simulink model "Helicopter_Sim"  (Simulink 8.6)
settings: Solver=ode4  StartTime=0.0  StopTime=Simulation_Tmax  FixedStep=Simulation_DT  RelTol=1e-3
values from neighbouring files (symbols this model uses):
  Disturbance_mass = 0    [Helicopter_EqPts.m]    (also in Helicopter_Params.m = 70)
  gravity = 9.81    [Helicopter_EqPts.m]    (also in Helicopter_Params.m)
  Helicopter_Fuselage_Area = 2    [Helicopter_EqPts.m]    (also in Helicopter_Params.m = 200)
  Helicopter_Fuselage_DragCoefficient = 15    [Helicopter_EqPts.m]    (also in Helicopter_Params.m = 40)
  Helicopter_Fuselage_Mass = 5    [Helicopter_EqPts.m]    (also in Helicopter_Params.m = 1000)
  Helicopter_Fuselage_RotInertia = 50    [Helicopter_EqPts.m]    (also in Helicopter_Params.m = 5)
  Helicopter_mRotor_Area = pi*Helicopter_mRotor_Radius^2    (= 3.14159265359)    [Helicopter_EqPts.m]    (also in Helicopter_Params.m = 314.159265359)
  Helicopter_mRotor_Ib = 10    [Helicopter_EqPts.m]    (also in Helicopter_Params.m)
  Helicopter_mRotor_Omega = 10    [Helicopter_EqPts.m]    (also in Helicopter_Params.m)
  Helicopter_mRotor_Radius = 1    [Helicopter_EqPts.m]    (also in Helicopter_Params.m = 10)
  Helicopter_N = 3    [Helicopter_EqPts.m]    (also in Helicopter_Params.m)
  Helicopter_tDistance = 3    [Helicopter_EqPts.m]    (also in Helicopter_Params.m = 20)
  Helicopter_tRotor_Area = pi*Helicopter_tRotor_Radius^2    (= 0.785398163397)    [Helicopter_EqPts.m]    (also in Helicopter_Params.m = 7853.98163397)
  Helicopter_tRotor_Radius = 0.5    [Helicopter_EqPts.m]    (also in Helicopter_Params.m = 50)
  Omega_Tail = -0.002043    [Helicopter_Params.m]
  rho_air = 1.22    [Helicopter_EqPts.m]    (also in Helicopter_Params.m)
  Simulation_DT = 0.00125    [Helicopter_EqPts.m]    (also in Helicopter_Params.m = 0.0125)
  Theta = 0.001706    [Helicopter_Params.m]
settings Model: Creator=Dana  LastModifiedBy=dmartin_a
settings DataIOCC: ExternalInput=[Helicopter, Disturbance, Simulation, gravity, rho_air]  InitialState=[Initial.Z ;Initial.R;]  SignalLoggingSaveFormat=Dataset  ReturnWorkspaceOutputs=on
settings OptimizationCC: ExpressionDepthLimit=128
settings DebuggingCC: UnderspecifiedInitializationDetection=Simplified  MergeDetectMultiDrivingBlocksExec=error  SolverPrmCheckMsg=none  FcnCallInpInsideContextMsg=EnableAllAsError  StateNameClashWarn=none  InitInArrayFormatMsg=error
settings GRTTargetCC: CombineOutputUpdateFcns=on  GRTInterface=off

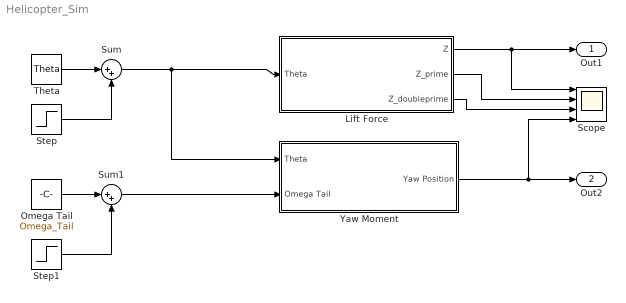
== system Helicopter_Sim ==
  Lift Force : Subsystem
  Omega Tail : Constant  Value=Omega_Tail  SampleTime=Simulation_DT
  Scope : Scope  NumInputPorts=4
  Step : Step  SampleTime=Simulation_DT
  Step1 : Step  SampleTime=Simulation_DT
  Sum : Sum  Inputs=|++
  Sum1 : Sum  Inputs=|++
  Theta : Constant  Value=Theta  SampleTime=Simulation_DT
  Yaw Moment : Subsystem
  Out1 : Outport
  Out2 : Outport  Port=2
  wires:
  Lift Force/1(Z) -> Scope/1, Out1/1
  Yaw Moment/1(Yaw Position) -> Scope/4, Out2/1
  Step/1 -> Sum/2
  Sum/1 -> Yaw Moment/1(Theta), Lift Force/1(Theta)
  Step1/1 -> Sum1/2
  Omega Tail/1 -> Sum1/1
  Sum1/1 -> Yaw Moment/2(Omega Tail)
  Theta/1 -> Sum/1
  Lift Force/2(Z_prime) -> Scope/2
  Lift Force/3(Z_doubleprime) -> Scope/3

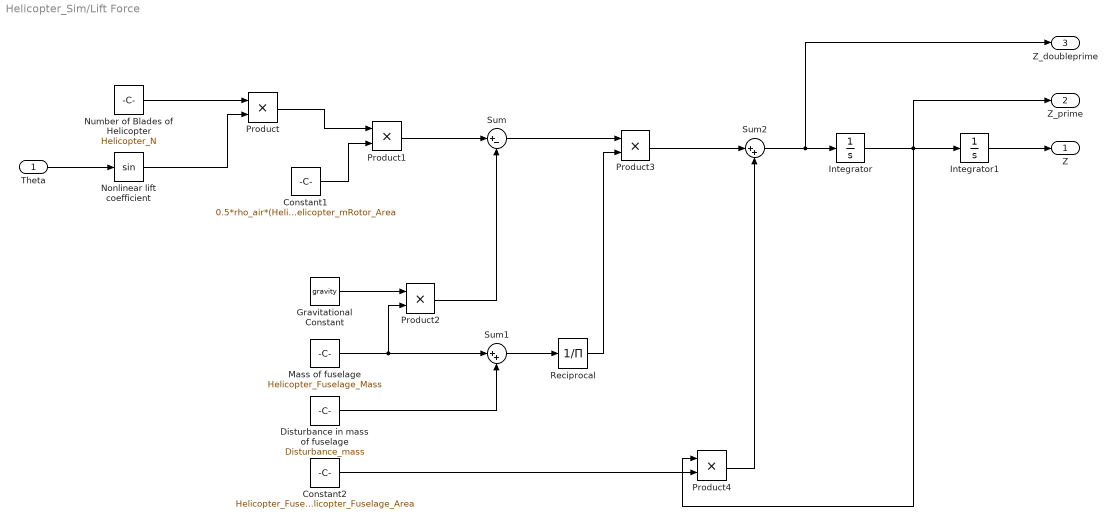
== system Helicopter_Sim/Lift Force ==
  Theta : Inport
  Constant1 : Constant  Value=0.5*rho_air*(Helicopter_mRotor_Omega*Helicopter_mRotor_Radius)^2*Helicopter_mRotor_Area  SampleTime=Simulation_DT
  Constant2 : Constant  Value=Helicopter_Fuselage_DragCoefficient*0.5*rho_air*Helicopter_Fuselage_Area  SampleTime=Simulation_DT
  Disturbance in mass of fuselage : Constant  Value=Disturbance_mass  SampleTime=Simulation_DT
  Gravitational Constant : Constant  Value=gravity  SampleTime=Simulation_DT
  Integrator : Integrator  LimitOutput=on  UpperSaturationLimit=20  LowerSaturationLimit=0
  Integrator1 : Integrator  LimitOutput=on  UpperSaturationLimit=20  LowerSaturationLimit=0
  Mass of fuselage : Constant  Value=Helicopter_Fuselage_Mass  SampleTime=Simulation_DT
  Nonlinear lift coefficient : Trigonometry  OutputSignalType=real
  Number of Blades of Helicopter : Constant  Value=Helicopter_N  SampleTime=Simulation_DT
  Product{,1..4} (5 alike) : Product
  Reciprocal : Product  Inputs=/  SaturateOnIntegerOverflow=on  RndMeth=Zero
  Sum : Sum  Inputs=|+-
  Sum1 : Sum  Inputs=|++
  Sum2 : Sum  Inputs=|++
  Z : Outport
  Z_prime : Outport  Port=2
  Z_doubleprime : Outport  Port=3
  wires:
  Theta/1 -> Nonlinear lift coefficient/1
  Number of Blades of Helicopter/1 -> Product/1
  Nonlinear lift coefficient/1 -> Product/2
  Product/1 -> Product1/1
  Constant1/1 -> Product1/2
  Mass of fuselage/1 -> Product2/2, Sum1/1
  Gravitational Constant/1 -> Product2/1
  Product2/1 -> Sum/2
  Product1/1 -> Sum/1
  Disturbance in mass of fuselage/1 -> Sum1/2
  Sum1/1 -> Reciprocal/1
  Reciprocal/1 -> Product3/2
  Sum/1 -> Product3/1
  Product3/1 -> Sum2/1
  Constant2/1 -> Product4/2
  Product4/1 -> Sum2/2
  Sum2/1 -> Z_doubleprime/1, Integrator/1
  Integrator/1 -> Z_prime/1, Integrator1/1, Product4/1
  Integrator1/1 -> Z/1

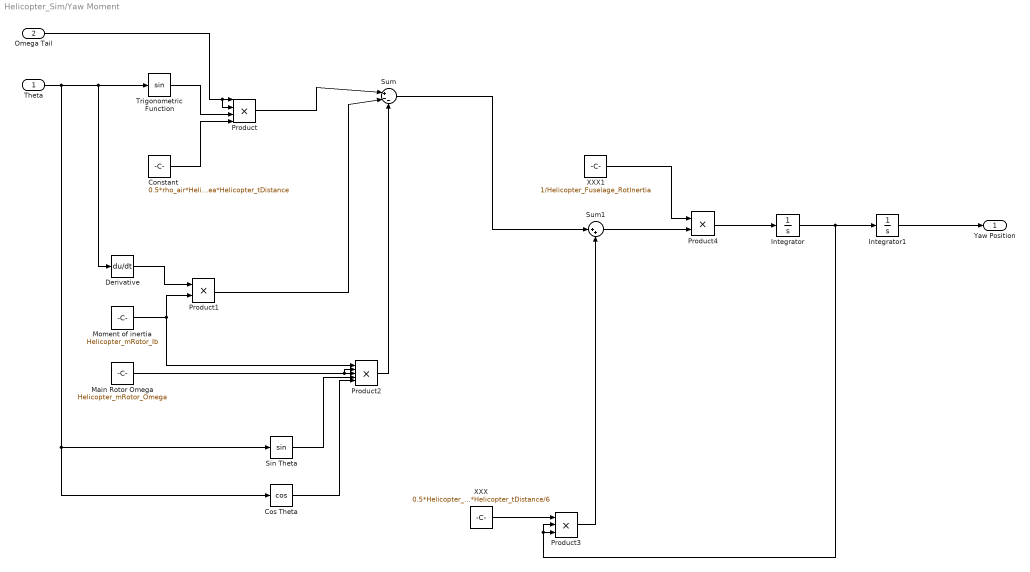
== system Helicopter_Sim/Yaw Moment ==
  Theta : Inport
  Omega Tail : Inport  Port=2
  Constant : Constant  Value=0.5*rho_air*Helicopter_tRotor_Radius^2*Helicopter_tRotor_Area*Helicopter_tDistance  SampleTime=Simulation_DT
  Cos Theta : Trigonometry  Operator=cos
  Derivative : Derivative
  Integrator : Integrator  LimitOutput=on  UpperSaturationLimit=20  LowerSaturationLimit=0
  Integrator1 : Integrator  LimitOutput=on  UpperSaturationLimit=20  LowerSaturationLimit=0
  Main Rotor Omega : Constant  Value=Helicopter_mRotor_Omega  SampleTime=Simulation_DT
  Moment of inertia : Constant  Value=Helicopter_mRotor_Ib  SampleTime=Simulation_DT
  Product : Product  Inputs=4
  Product1 : Product
  Product2 : Product  Inputs=5
  Product3 : Product  Inputs=3
  Product4 : Product
  Sin Theta : Trigonometry
  Sum : Sum  Inputs=|+--
  Sum1 : Sum  Inputs=|++
  Trigonometric Function : Trigonometry
  XXX : Constant  Value=0.5*Helicopter_Fuselage_DragCoefficient*rho_air*2*Helicopter_Fuselage_Area*Helicopter_tDistance/6  SampleTime=Simulation_DT
  XXX1 : Constant  Value=1/Helicopter_Fuselage_RotInertia  SampleTime=Simulation_DT
  Yaw Position : Outport
  wires:
  Theta/1 -> Cos Theta/1, Sin Theta/1, Derivative/1, Trigonometric Function/1
  Product/1 -> Sum/1
  Moment of inertia/1 -> Product1/2, Product2/1
  Derivative/1 -> Product1/1
  Product1/1 -> Sum/2
  Main Rotor Omega/1 -> Product2/3, Product2/2
  Sin Theta/1 -> Product2/4
  Cos Theta/1 -> Product2/5
  Product2/1 -> Sum/3
  Trigonometric Function/1 -> Product/3
  Constant/1 -> Product/4
  Omega Tail/1 -> Product/2, Product/1
  Sum/1 -> Sum1/1
  Product3/1 -> Sum1/2
  Sum1/1 -> Product4/2
  XXX1/1 -> Product4/1
  Product4/1 -> Integrator/1
  Integrator1/1 -> Yaw Position/1
  Integrator/1 -> Integrator1/1, Product3/3, Product3/2
  XXX/1 -> Product3/1
